simulink library "carnotUIBK"  (R2018b)
settings: Solver=VariableStepAuto  StartTime=0.0  StopTime=10.0  RelTol=1e-3  EnableMultiTasking=on
values from neighbouring files (symbols this model uses):
  A = 7*10*2    (= 140)    [theta_ground_v1.m]    (also in xlswrite1.m = num2cell(data))
  amb_factor = 1    [DOOR.m]    (also in WALL.m; WINDOW.m = 0)
  area = obj.width * obj.height    [DOOR.m]    (also in RES.m = []; ROOM.m = 0; THERMALZONE.m = area + room(kk).area; WALL.m = area - obj.doors(jj).calc_area())
  B = A/(0.5 * P)    (= 8.23529411765)    [theta_ground_v1.m]
  boundary = BOUNDARY()    [BUILDING.m]    (also in WALL.m = '')
  building = obj    [BUILDING.m]    (also in create_building_automatic.m = building.save(); ini_building_automatic.m = building.add_variant_hvac(building.variant_hvac, hvac); load_building_automatic.m = building.save())
  C = zeros(1,length(d)+1)    [CONSTRUCTION.m]    (also in DOOR.m = [0 0 0]; WALL.m = [0 0 0]; WINDOW.m = [0 0 0])
  control = 2    [GAIN.m]    (also in GAINS.m)
  cp = str2num(value)    [CONSTRUCTION.m]
  height = 0    [DOOR.m]    (also in ROOM.m; THERMALZONE.m; WALL.m; WINDOW.m)
  p = [timevec_weather weather(:,12)]    [BOUNDARY.m]    (also in WEATHER.m = 0; init_carnotUIBK.m = cell2mat(carnotUIBKpaths(i,2)))
  rho = str2num(value)    [CONSTRUCTION.m]    (also in theta_ground_v1.m = 2000)
  type = 1    [CONSTRUCTION.m]    (also in GAINS.m = raw_moisture{ii,3}; STRUCTURE.m = 0)
  view_factor = 1    [DOOR.m]    (also in WINDOW.m = 0)
  wall = []    [ROOM.m]
  z = obj.Z    [WALL.m]    (also in theta_ground_v1.m = 0)
  zone = obj.zone(ind)    [THERMALZONE.m]
undefined symbols (not defined in the file or in its folder): const, Dd, get_building, pos, Qdot_C, Qdot_H, Qdot_I_electricity, Qdot_I_light, Qdot_I_person, Qdot_S, Qdot_T_ground, Qdot_T_neighbour, Qdot_T_opaque, Qdot_T_window, Qdot_V_infiltration, Qdot_V_mech, Qdot_V_window, r_frame, solar_ratio, solar_ratio1, solar_ratio2, Tc, Tr, Ts, Uvalue, wallsurface, window, window_height, window_heigth, window_width, windowsurface, x_CO2, x_H2O, x_VOC
libraries: carnot x104, simulink x16, $bdroot x16, simulink_extras x14
(part 9 of 12)

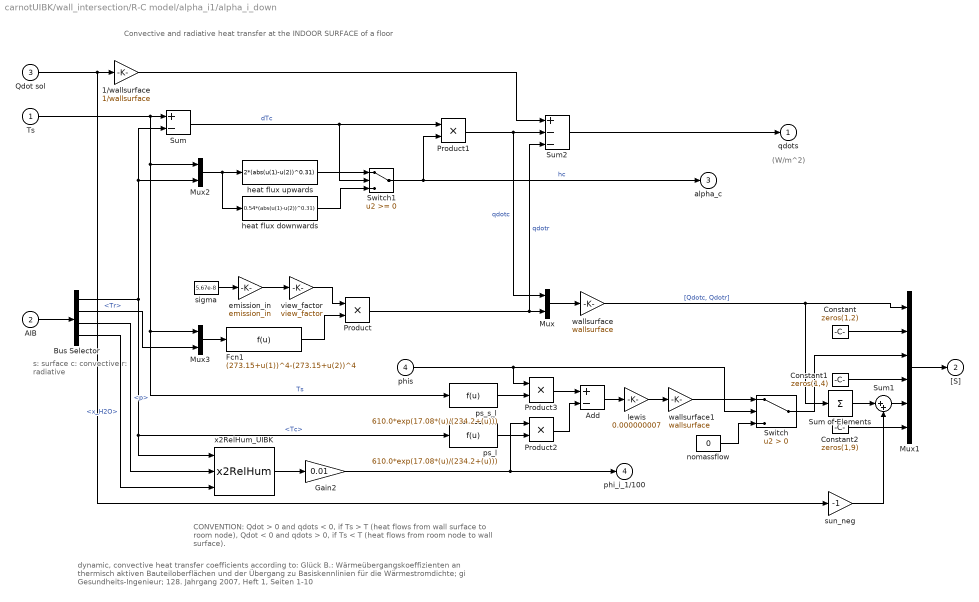
== system carnotUIBK/wall_intersection/R-C model/alpha_i1/alpha_i_down ==
  note: dynamic, convective heat transfer coefficients according to: Glück B.: Wärmeübergangskoeffizienten an thermisch aktiven Bauteiloberflächen
      | und der Übergang zu Basiskennlinien für die Wärmestromdichte; gi Gesundheits-Ingenieur; 128. Jahrgang 2007, Heft 1, Seiten 1-10
  note: s: surface
      | c: convective
      | r: radiative
  note: CONVENTION:
      | Qdot > 0 and qdots < 0, if Ts > T (heat flows from wall surface to room node),
      | Qdot < 0 and qdots > 0, if Ts < T (heat flows from room node to wall surface).
  note: Convective and radiative heat transfer at the INDOOR SURFACE of a floor
  note: (W/m^2)
  Ts : Inport
  AIB : Inport  Port=2
  Qdot sol : Inport  Port=3
  phis : Inport  Port=4
  1/wallsurface : Gain  Gain=1/wallsurface  SaturateOnIntegerOverflow=on  OutDataTypeStr=Inherit: Same as input  ParamDataTypeStr=Inherit: Same as input
  Add : Sum  Inputs=+-
  Bus Selector : BusSelector  OutputSignals=Tc,Tr,p,x_H2O
  Constant : Constant  Value=zeros(1,2)
  Constant1 : Constant  Value=zeros(1,4)
  Constant2 : Constant  Value=zeros(1,9)
  Fcn1 : Fcn  Expr=(273.15+u(1))^4-(273.15+u(2))^4
  Gain2 : Gain  Gain=0.01
  Mux : Mux  Inputs=2
  Mux1 : Mux  Inputs=[2 2 1 4 1 9]
  Mux2 : Mux  Inputs=2
  Mux3 : Mux  Inputs=2
  Product : Product  SaturateOnIntegerOverflow=on  RndMeth=Zero  InputSameDT=on  OutDataTypeStr=Inherit: Same as first input
  Product1 : Product  SaturateOnIntegerOverflow=on  RndMeth=Zero  InputSameDT=on  OutDataTypeStr=Inherit: Same as first input
  Product2 : Product  RndMeth=Zero
  Product3 : Product  RndMeth=Zero
  Sum : Sum  Inputs=+-  SaturateOnIntegerOverflow=on  InputSameDT=on  OutDataTypeStr=Inherit: Same as first input
  Sum of Elements : Sum  Inputs=+
  Sum1 : Sum  Inputs=|++
  Sum2 : Sum  Inputs=+--  SaturateOnIntegerOverflow=on  InputSameDT=on  OutDataTypeStr=Inherit: Same as first input
  Switch : Switch  Criteria=u2 > Threshold
  Switch1 : Switch
  emission_in : Gain  Gain=emission_in  SaturateOnIntegerOverflow=on  OutDataTypeStr=Inherit: Same as input  ParamDataTypeStr=Inherit: Same as input
  heat flux downwards : Fcn  Expr=0.54*(abs(u(1)-u(2))^0.31)
  heat flux upwards : Fcn  Expr=2*(abs(u(1)-u(2))^0.31)
  lewis : Gain  Gain=0.000000007  SaturateOnIntegerOverflow=on  OutDataTypeStr=Inherit: Same as input  ParamDataTypeStr=Inherit: Same as input
  nomassflow : Constant  Value=0
  ps_l : Fcn  Expr=610.0*exp(17.08*(u)/(234.2+(u)))
  ps_s_l : Fcn  Expr=610.0*exp(17.08*(u)/(234.2+(u)))
  sigma : Constant  Value=5.67e-8
  sun_neg : Gain  Gain=-1  SaturateOnIntegerOverflow=on  OutDataTypeStr=Inherit: Same as input  ParamDataTypeStr=Inherit: Same as input
  view_factor : Gain  Gain=view_factor  SaturateOnIntegerOverflow=on  OutDataTypeStr=Inherit: Same as input  ParamDataTypeStr=Inherit: Same as input
  wallsurface : Gain  Gain=wallsurface  SaturateOnIntegerOverflow=on  OutDataTypeStr=Inherit: Same as input  ParamDataTypeStr=Inherit: Same as input
  wallsurface1 : Gain  Gain=wallsurface  SaturateOnIntegerOverflow=on  OutDataTypeStr=Inherit: Same as input  ParamDataTypeStr=Inherit: Same as input
  x2RelHum_UIBK : carnot/Basic/Material_Properties/x2RelHum
  qdots : Outport  InitialOutput=0
  "[S]" : Outport  Port=2  InitialOutput=0
  alpha_c : Outport  Port=3  InitialOutput=0
  phi_i_1/100 : Outport  Port=4  InitialOutput=0
  wires:
  heat flux downwards/1 -> Switch1/3
  heat flux upwards/1 -> Switch1/1
  Sum/1 -> Product1/1, Switch1/2  "dTc"
  1/wallsurface/1 -> Sum2/1
  wallsurface/1 -> Sum of Elements/1, Mux1/1  "[Qdotc, Qdotr]"
  Switch1/1 -> alpha_c/1, Product1/2  "hc"
  Product1/1 -> Sum2/2, Mux/1  "qdotc"
  Mux2/1 -> heat flux upwards/1, heat flux downwards/1
  Bus Selector/2 -> Mux3/2  "<Tr>"
  Ts/1 -> Mux2/1, Mux3/1, ps_s_l/1, Sum/1  "Ts"
  Mux/1 -> wallsurface/1
  Product/1 -> Mux/2, Sum2/3  "qdotr"
  emission_in/1 -> view_factor/1
  Bus Selector/1 -> x2RelHum_UIBK/1, ps_l/1, Mux2/2, Sum/2  "<Tc>"
  AIB/1 -> Bus Selector/1
  Sum2/1 -> qdots/1
  Mux1/1 -> "[S]"/1
  sigma/1 -> emission_in/1
  Mux3/1 -> Fcn1/1
  Fcn1/1 -> Product/2
  x2RelHum_UIBK/1 -> Gain2/1
  Bus Selector/3 -> x2RelHum_UIBK/2  "<p>"
  Bus Selector/4 -> x2RelHum_UIBK/3  "<x_H2O>"
  Gain2/1 -> phi_i_1/100/1, Product2/1
  lewis/1 -> wallsurface1/1
  Constant2/1 -> Mux1/6
  Constant1/1 -> Mux1/4
  Constant/1 -> Mux1/2
  ps_l/1 -> Product2/2
  ps_s_l/1 -> Product3/2
  Product3/1 -> Add/1
  Product2/1 -> Add/2
  Add/1 -> lewis/1
  phis/1 -> Switch/2, Product3/1
  view_factor/1 -> Product/1
  wallsurface1/1 -> Switch/1
  Switch/1 -> Mux1/3
  nomassflow/1 -> Switch/3
  Sum1/1 -> Mux1/5
  Sum of Elements/1 -> Sum1/1
  Qdot sol/1 -> 1/wallsurface/1, sun_neg/1
  sun_neg/1 -> Sum1/2

== system carnotUIBK/wall_intersection/R-C model/alpha_i1/alpha_i_horizontal ==
  note: dynamic, convective heat transfer coefficients according to: Glück B.: Wärmeübergangskoeffizienten an thermisch aktiven Bauteiloberflächen
      | und der Übergang zu Basiskennlinien für die Wärmestromdichte; gi Gesundheits-Ingenieur; 128. Jahrgang 2007, Heft 1, Seiten 1-10
  note: s: surface
      | c: convective
      | r: radiative
  note: CONVENTION:
      | Qdot > 0 and qdots < 0, if Ts > T (heat flows from wall surface to room node),
      | Qdot < 0 and qdots > 0, if Ts < T (heat flows from room node to wall surface).
  note: Convective and radiative heat transfer at the INDOOR SURFACE of a VERTICAL OUTER WALL
  note: (W/m^2)
  Ts : Inport
  AIB : Inport  Port=2
  Qdot sol : Inport  Port=3
  phis : Inport  Port=4
  1/wallsurface : Gain  Gain=1/wallsurface  SaturateOnIntegerOverflow=on  OutDataTypeStr=Inherit: Same as input  ParamDataTypeStr=Inherit: Same as input
  Add : Sum  Inputs=+-
  Bus Selector : BusSelector  OutputSignals=Tc,Tr,p,x_H2O
  Constant : Constant  Value=zeros(1,2)
  Constant4 : Constant  Value=zeros(1,4)
  Constant5 : Constant  Value=zeros(1,9)
  Fcn : Fcn  Expr=1.6*(abs(u(1)-u(2)))^0.3
  Fcn1 : Fcn  Expr=(273.15+u(1))^4-(273.15+u(2))^4
  Gain2 : Gain  Gain=0.01
  Mux : Mux  Inputs=2
  Mux2 : Mux  Inputs=2
  Mux3 : Mux  Inputs=2
  Mux4 : Mux  Inputs=[2 2 1 4 1 9]
  Product : Product  SaturateOnIntegerOverflow=on  RndMeth=Zero  InputSameDT=on  OutDataTypeStr=Inherit: Same as first input
  Product1 : Product  SaturateOnIntegerOverflow=on  RndMeth=Zero  InputSameDT=on  OutDataTypeStr=Inherit: Same as first input
  Product2 : Product  RndMeth=Zero
  Product3 : Product  RndMeth=Zero
  Sum : Sum  Inputs=+-  SaturateOnIntegerOverflow=on  InputSameDT=on  OutDataTypeStr=Inherit: Same as first input
  Sum of Elements : Sum  Inputs=+
  Sum1 : Sum  Inputs=|++
  Sum2 : Sum  Inputs=+--  SaturateOnIntegerOverflow=on  InputSameDT=on  OutDataTypeStr=Inherit: Same as first input
  Switch : Switch  Criteria=u2 > Threshold
  emission_in : Gain  Gain=emission_in  SaturateOnIntegerOverflow=on  OutDataTypeStr=Inherit: Same as input  ParamDataTypeStr=Inherit: Same as input
  lewis : Gain  Gain=0.000000007  SaturateOnIntegerOverflow=on  OutDataTypeStr=Inherit: Same as input  ParamDataTypeStr=Inherit: Same as input
  nomassflow : Constant  Value=0
  ps_l : Fcn  Expr=610.0*exp(17.08*(u)/(234.2+(u)))
  ps_s_l : Fcn  Expr=610.0*exp(17.08*(u)/(234.2+(u)))
  sigma : Constant  Value=5.67e-8
  sun_neg : Gain  Gain=-1  SaturateOnIntegerOverflow=on  OutDataTypeStr=Inherit: Same as input  ParamDataTypeStr=Inherit: Same as input
  view_factor : Gain  Gain=view_factor  SaturateOnIntegerOverflow=on  OutDataTypeStr=Inherit: Same as input  ParamDataTypeStr=Inherit: Same as input
  wallsurface : Gain  Gain=wallsurface  SaturateOnIntegerOverflow=on  OutDataTypeStr=Inherit: Same as input  ParamDataTypeStr=Inherit: Same as input
  wallsurface1 : Gain  Gain=wallsurface  SaturateOnIntegerOverflow=on  OutDataTypeStr=Inherit: Same as input  ParamDataTypeStr=Inherit: Same as input
  x2RelHum_UIBK : carnot/Basic/Material_Properties/x2RelHum
  qdots : Outport  InitialOutput=0
  "[S]" : Outport  Port=2  InitialOutput=0
  alpha_c : Outport  Port=3  InitialOutput=0
  phi_i_1/100 : Outport  Port=4  InitialOutput=0
  wires:
  1/wallsurface/1 -> Sum2/1
  Qdot sol/1 -> sun_neg/1, 1/wallsurface/1
  wallsurface/1 -> Sum of Elements/1, Mux4/1  "[Qdotc, Qdotr]"
  Fcn/1 -> Product1/2, alpha_c/1  "hc"
  Product1/1 -> Sum2/2, Mux/1  "qdotc"
  Mux2/1 -> Fcn/1
  Bus Selector/2 -> Mux3/2  "<Tr>"
  Sum/1 -> Product1/1  "dTc"
  Ts/1 -> Mux2/1, Mux3/1, ps_s_l/1, Sum/1  "Ts"
  Mux/1 -> wallsurface/1
  Product/1 -> Mux/2, Sum2/3  "qdotr"
  emission_in/1 -> view_factor/1
  Bus Selector/1 -> x2RelHum_UIBK/1, ps_l/1, Mux2/2, Sum/2  "<Tc>"
  AIB/1 -> Bus Selector/1
  Sum2/1 -> qdots/1
  Mux4/1 -> "[S]"/1
  sigma/1 -> emission_in/1
  Mux3/1 -> Fcn1/1
  Fcn1/1 -> Product/2
  x2RelHum_UIBK/1 -> Gain2/1
  Bus Selector/3 -> x2RelHum_UIBK/2  "<p>"
  Bus Selector/4 -> x2RelHum_UIBK/3  "<x_H2O>"
  Gain2/1 -> phi_i_1/100/1, Product2/1
  lewis/1 -> wallsurface1/1
  ps_l/1 -> Product2/2
  ps_s_l/1 -> Product3/2
  Product3/1 -> Add/1
  Product2/1 -> Add/2
  Add/1 -> lewis/1
  phis/1 -> Switch/2, Product3/1
  view_factor/1 -> Product/1
  wallsurface1/1 -> Switch/1
  Switch/1 -> Mux4/3
  nomassflow/1 -> Switch/3
  Constant/1 -> Mux4/2
  Constant5/1 -> Mux4/6
  Constant4/1 -> Mux4/4
  Sum1/1 -> Mux4/5
  Sum of Elements/1 -> Sum1/1
  sun_neg/1 -> Sum1/2

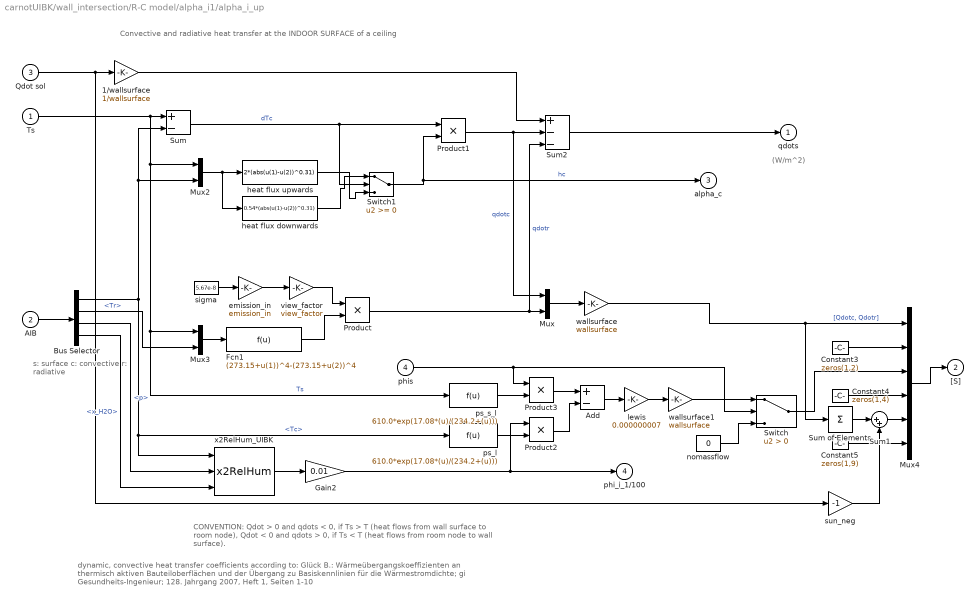
== system carnotUIBK/wall_intersection/R-C model/alpha_i1/alpha_i_up ==
  note: dynamic, convective heat transfer coefficients according to: Glück B.: Wärmeübergangskoeffizienten an thermisch aktiven Bauteiloberflächen
      | und der Übergang zu Basiskennlinien für die Wärmestromdichte; gi Gesundheits-Ingenieur; 128. Jahrgang 2007, Heft 1, Seiten 1-10
  note: s: surface
      | c: convective
      | r: radiative
  note: CONVENTION:
      | Qdot > 0 and qdots < 0, if Ts > T (heat flows from wall surface to room node),
      | Qdot < 0 and qdots > 0, if Ts < T (heat flows from room node to wall surface).
  note: Convective and radiative heat transfer at the INDOOR SURFACE of a ceiling
  note: (W/m^2)
  Ts : Inport
  AIB : Inport  Port=2
  Qdot sol : Inport  Port=3
  phis : Inport  Port=4
  1/wallsurface : Gain  Gain=1/wallsurface  SaturateOnIntegerOverflow=on  OutDataTypeStr=Inherit: Same as input  ParamDataTypeStr=Inherit: Same as input
  Add : Sum  Inputs=+-
  Bus Selector : BusSelector  OutputSignals=Tc,Tr,p,x_H2O
  Constant3 : Constant  Value=zeros(1,2)
  Constant4 : Constant  Value=zeros(1,4)
  Constant5 : Constant  Value=zeros(1,9)
  Fcn1 : Fcn  Expr=(273.15+u(1))^4-(273.15+u(2))^4
  Gain2 : Gain  Gain=0.01
  Mux : Mux  Inputs=2
  Mux2 : Mux  Inputs=2
  Mux3 : Mux  Inputs=2
  Mux4 : Mux  Inputs=[2 2 1 4 1 9]
  Product : Product  SaturateOnIntegerOverflow=on  RndMeth=Zero  InputSameDT=on  OutDataTypeStr=Inherit: Same as first input
  Product1 : Product  SaturateOnIntegerOverflow=on  RndMeth=Zero  InputSameDT=on  OutDataTypeStr=Inherit: Same as first input
  Product2 : Product  RndMeth=Zero
  Product3 : Product  RndMeth=Zero
  Sum : Sum  Inputs=+-  SaturateOnIntegerOverflow=on  InputSameDT=on  OutDataTypeStr=Inherit: Same as first input
  Sum of Elements : Sum  Inputs=+
  Sum1 : Sum  Inputs=|++
  Sum2 : Sum  Inputs=+--  SaturateOnIntegerOverflow=on  InputSameDT=on  OutDataTypeStr=Inherit: Same as first input
  Switch : Switch  Criteria=u2 > Threshold
  Switch1 : Switch
  emission_in : Gain  Gain=emission_in  SaturateOnIntegerOverflow=on  OutDataTypeStr=Inherit: Same as input  ParamDataTypeStr=Inherit: Same as input
  heat flux downwards : Fcn  Expr=0.54*(abs(u(1)-u(2))^0.31)
  heat flux upwards : Fcn  Expr=2*(abs(u(1)-u(2))^0.31)
  lewis : Gain  Gain=0.000000007  SaturateOnIntegerOverflow=on  OutDataTypeStr=Inherit: Same as input  ParamDataTypeStr=Inherit: Same as input
  nomassflow : Constant  Value=0
  ps_l : Fcn  Expr=610.0*exp(17.08*(u)/(234.2+(u)))
  ps_s_l : Fcn  Expr=610.0*exp(17.08*(u)/(234.2+(u)))
  sigma : Constant  Value=5.67e-8
  sun_neg : Gain  Gain=-1  SaturateOnIntegerOverflow=on  OutDataTypeStr=Inherit: Same as input  ParamDataTypeStr=Inherit: Same as input
  view_factor : Gain  Gain=view_factor  SaturateOnIntegerOverflow=on  OutDataTypeStr=Inherit: Same as input  ParamDataTypeStr=Inherit: Same as input
  wallsurface : Gain  Gain=wallsurface  SaturateOnIntegerOverflow=on  OutDataTypeStr=Inherit: Same as input  ParamDataTypeStr=Inherit: Same as input
  wallsurface1 : Gain  Gain=wallsurface  SaturateOnIntegerOverflow=on  OutDataTypeStr=Inherit: Same as input  ParamDataTypeStr=Inherit: Same as input
  x2RelHum_UIBK : carnot/Basic/Material_Properties/x2RelHum
  qdots : Outport  InitialOutput=0
  "[S]" : Outport  Port=2  InitialOutput=0
  alpha_c : Outport  Port=3  InitialOutput=0
  phi_i_1/100 : Outport  Port=4  InitialOutput=0
  wires:
  heat flux downwards/1 -> Switch1/1
  heat flux upwards/1 -> Switch1/3
  Sum/1 -> Product1/1, Switch1/2  "dTc"
  1/wallsurface/1 -> Sum2/1
  Qdot sol/1 -> sun_neg/1, 1/wallsurface/1
  Switch1/1 -> alpha_c/1, Product1/2  "hc"
  Product1/1 -> Sum2/2, Mux/1  "qdotc"
  Mux2/1 -> heat flux upwards/1, heat flux downwards/1
  Bus Selector/2 -> Mux3/2  "<Tr>"
  Ts/1 -> Mux2/1, Mux3/1, ps_s_l/1, Sum/1  "Ts"
  Mux/1 -> wallsurface/1
  Product/1 -> Mux/2, Sum2/3  "qdotr"
  emission_in/1 -> view_factor/1
  Bus Selector/1 -> x2RelHum_UIBK/1, ps_l/1, Mux2/2, Sum/2  "<Tc>"
  AIB/1 -> Bus Selector/1
  Sum2/1 -> qdots/1
  sigma/1 -> emission_in/1
  Mux3/1 -> Fcn1/1
  Fcn1/1 -> Product/2
  x2RelHum_UIBK/1 -> Gain2/1
  Bus Selector/3 -> x2RelHum_UIBK/2  "<p>"
  Bus Selector/4 -> x2RelHum_UIBK/3  "<x_H2O>"
  Gain2/1 -> phi_i_1/100/1, Product2/1
  lewis/1 -> wallsurface1/1
  ps_l/1 -> Product2/2
  ps_s_l/1 -> Product3/2
  Product3/1 -> Add/1
  Product2/1 -> Add/2
  Add/1 -> lewis/1
  phis/1 -> Switch/2, Product3/1
  view_factor/1 -> Product/1
  wallsurface1/1 -> Switch/1
  Switch/1 -> Mux4/3
  nomassflow/1 -> Switch/3
  wallsurface/1 -> Sum of Elements/1, Mux4/1  "[Qdotc, Qdotr]"
  Mux4/1 -> "[S]"/1
  Constant5/1 -> Mux4/6
  Constant4/1 -> Mux4/4
  Constant3/1 -> Mux4/2
  Sum of Elements/1 -> Sum1/1
  Sum1/1 -> Mux4/5
  sun_neg/1 -> Sum1/2

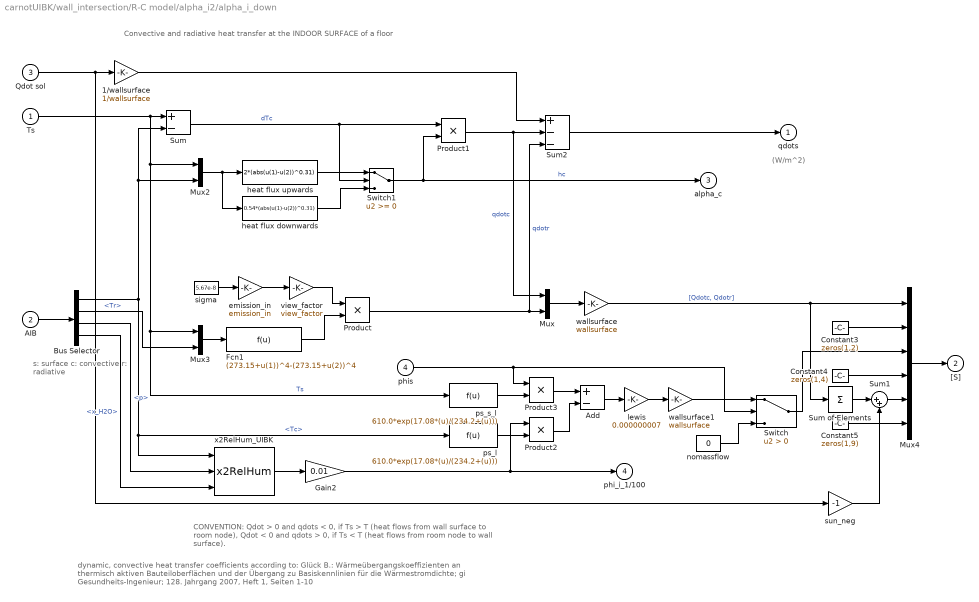
== system carnotUIBK/wall_intersection/R-C model/alpha_i2/alpha_i_down ==
  note: (W/m^2)
  note: Convective and radiative heat transfer at the INDOOR SURFACE of a floor
  note: CONVENTION:
      | Qdot > 0 and qdots < 0, if Ts > T (heat flows from wall surface to room node),
      | Qdot < 0 and qdots > 0, if Ts < T (heat flows from room node to wall surface).
  note: s: surface
      | c: convective
      | r: radiative
  note: dynamic, convective heat transfer coefficients according to: Glück B.: Wärmeübergangskoeffizienten an thermisch aktiven Bauteiloberflächen
      | und der Übergang zu Basiskennlinien für die Wärmestromdichte; gi Gesundheits-Ingenieur; 128. Jahrgang 2007, Heft 1, Seiten 1-10
  Ts : Inport
  AIB : Inport  Port=2
  Qdot sol : Inport  Port=3
  phis : Inport  Port=4
  1/wallsurface : Gain  Gain=1/wallsurface  SaturateOnIntegerOverflow=on  OutDataTypeStr=Inherit: Same as input  ParamDataTypeStr=Inherit: Same as input
  Add : Sum  Inputs=+-
  Bus Selector : BusSelector  OutputSignals=Tc,Tr,p,x_H2O
  Constant3 : Constant  Value=zeros(1,2)
  Constant4 : Constant  Value=zeros(1,4)
  Constant5 : Constant  Value=zeros(1,9)
  Fcn1 : Fcn  Expr=(273.15+u(1))^4-(273.15+u(2))^4
  Gain2 : Gain  Gain=0.01
  Mux : Mux  Inputs=2
  Mux2 : Mux  Inputs=2
  Mux3 : Mux  Inputs=2
  Mux4 : Mux  Inputs=[2 2 1 4 1 9]
  Product : Product  SaturateOnIntegerOverflow=on  RndMeth=Zero  InputSameDT=on  OutDataTypeStr=Inherit: Same as first input
  Product1 : Product  SaturateOnIntegerOverflow=on  RndMeth=Zero  InputSameDT=on  OutDataTypeStr=Inherit: Same as first input
  Product2 : Product  RndMeth=Zero
  Product3 : Product  RndMeth=Zero
  Sum : Sum  Inputs=+-  SaturateOnIntegerOverflow=on  InputSameDT=on  OutDataTypeStr=Inherit: Same as first input
  Sum of Elements : Sum  Inputs=+
  Sum1 : Sum  Inputs=|++
  Sum2 : Sum  Inputs=+--  SaturateOnIntegerOverflow=on  InputSameDT=on  OutDataTypeStr=Inherit: Same as first input
  Switch : Switch  Criteria=u2 > Threshold
  Switch1 : Switch
  emission_in : Gain  Gain=emission_in  SaturateOnIntegerOverflow=on  OutDataTypeStr=Inherit: Same as input  ParamDataTypeStr=Inherit: Same as input
  heat flux downwards : Fcn  Expr=0.54*(abs(u(1)-u(2))^0.31)
  heat flux upwards : Fcn  Expr=2*(abs(u(1)-u(2))^0.31)
  lewis : Gain  Gain=0.000000007  SaturateOnIntegerOverflow=on  OutDataTypeStr=Inherit: Same as input  ParamDataTypeStr=Inherit: Same as input
  nomassflow : Constant  Value=0
  ps_l : Fcn  Expr=610.0*exp(17.08*(u)/(234.2+(u)))
  ps_s_l : Fcn  Expr=610.0*exp(17.08*(u)/(234.2+(u)))
  sigma : Constant  Value=5.67e-8
  sun_neg : Gain  Gain=-1  SaturateOnIntegerOverflow=on  OutDataTypeStr=Inherit: Same as input  ParamDataTypeStr=Inherit: Same as input
  view_factor : Gain  Gain=view_factor  SaturateOnIntegerOverflow=on  OutDataTypeStr=Inherit: Same as input  ParamDataTypeStr=Inherit: Same as input
  wallsurface : Gain  Gain=wallsurface  SaturateOnIntegerOverflow=on  OutDataTypeStr=Inherit: Same as input  ParamDataTypeStr=Inherit: Same as input
  wallsurface1 : Gain  Gain=wallsurface  SaturateOnIntegerOverflow=on  OutDataTypeStr=Inherit: Same as input  ParamDataTypeStr=Inherit: Same as input
  x2RelHum_UIBK : carnot/Basic/Material_Properties/x2RelHum
  qdots : Outport  InitialOutput=0
  "[S]" : Outport  Port=2  InitialOutput=0
  alpha_c : Outport  Port=3  InitialOutput=0
  phi_i_1/100 : Outport  Port=4  InitialOutput=0
  wires:
  nomassflow/1 -> Switch/3
  Switch/1 -> Mux4/3
  wallsurface1/1 -> Switch/1
  view_factor/1 -> Product/1
  phis/1 -> Product3/1, Switch/2
  Add/1 -> lewis/1
  Product2/1 -> Add/2
  Product3/1 -> Add/1
  ps_s_l/1 -> Product3/2
  ps_l/1 -> Product2/2
  lewis/1 -> wallsurface1/1
  Gain2/1 -> Product2/1, phi_i_1/100/1
  Bus Selector/4 -> x2RelHum_UIBK/3  "<x_H2O>"
  Bus Selector/3 -> x2RelHum_UIBK/2  "<p>"
  x2RelHum_UIBK/1 -> Gain2/1
  Fcn1/1 -> Product/2
  Mux3/1 -> Fcn1/1
  sigma/1 -> emission_in/1
  Mux4/1 -> "[S]"/1
  Sum2/1 -> qdots/1
  AIB/1 -> Bus Selector/1
  Bus Selector/1 -> Sum/2, Mux2/2, x2RelHum_UIBK/1, ps_l/1  "<Tc>"
  emission_in/1 -> view_factor/1
  Product/1 -> Sum2/3, Mux/2  "qdotr"
  Mux/1 -> wallsurface/1
  Ts/1 -> Sum/1, ps_s_l/1, Mux3/1, Mux2/1  "Ts"
  Bus Selector/2 -> Mux3/2  "<Tr>"
  Mux2/1 -> heat flux downwards/1, heat flux upwards/1
  Product1/1 -> Mux/1, Sum2/2  "qdotc"
  Switch1/1 -> Product1/2, alpha_c/1  "hc"
  wallsurface/1 -> Sum of Elements/1, Mux4/1  "[Qdotc, Qdotr]"
  Qdot sol/1 -> sun_neg/1, 1/wallsurface/1
  1/wallsurface/1 -> Sum2/1
  Sum/1 -> Switch1/2, Product1/1  "dTc"
  heat flux upwards/1 -> Switch1/1
  heat flux downwards/1 -> Switch1/3
  Constant5/1 -> Mux4/6
  Constant4/1 -> Mux4/4
  Constant3/1 -> Mux4/2
  Sum of Elements/1 -> Sum1/1
  Sum1/1 -> Mux4/5
  sun_neg/1 -> Sum1/2

== system carnotUIBK/wall_intersection/R-C model/alpha_i2/alpha_i_horizontal ==
  note: (W/m^2)
  note: Convective and radiative heat transfer at the INDOOR SURFACE of a VERTICAL OUTER WALL
  note: CONVENTION:
      | Qdot > 0 and qdots < 0, if Ts > T (heat flows from wall surface to room node),
      | Qdot < 0 and qdots > 0, if Ts < T (heat flows from room node to wall surface).
  note: s: surface
      | c: convective
      | r: radiative
  note: dynamic, convective heat transfer coefficients according to: Glück B.: Wärmeübergangskoeffizienten an thermisch aktiven Bauteiloberflächen
      | und der Übergang zu Basiskennlinien für die Wärmestromdichte; gi Gesundheits-Ingenieur; 128. Jahrgang 2007, Heft 1, Seiten 1-10
  Ts : Inport
  AIB : Inport  Port=2
  Qdot sol : Inport  Port=3
  phis : Inport  Port=4
  1/wallsurface : Gain  Gain=1/wallsurface  SaturateOnIntegerOverflow=on  OutDataTypeStr=Inherit: Same as input  ParamDataTypeStr=Inherit: Same as input
  Add : Sum  Inputs=+-
  Bus Selector : BusSelector  OutputSignals=Tc,Tr,p,x_H2O
  Constant3 : Constant  Value=zeros(1,2)
  Constant4 : Constant  Value=zeros(1,4)
  Constant5 : Constant  Value=zeros(1,9)
  Fcn : Fcn  Expr=1.6*(abs(u(1)-u(2)))^0.3
  Fcn1 : Fcn  Expr=(273.15+u(1))^4-(273.15+u(2))^4
  Gain2 : Gain  Gain=0.01
  Mux : Mux  Inputs=2
  Mux2 : Mux  Inputs=2
  Mux3 : Mux  Inputs=2
  Mux4 : Mux  Inputs=[2 2 1 4 1 9]
  Product : Product  SaturateOnIntegerOverflow=on  RndMeth=Zero  InputSameDT=on  OutDataTypeStr=Inherit: Same as first input
  Product1 : Product  SaturateOnIntegerOverflow=on  RndMeth=Zero  InputSameDT=on  OutDataTypeStr=Inherit: Same as first input
  Product2 : Product  RndMeth=Zero
  Product3 : Product  RndMeth=Zero
  Sum : Sum  Inputs=+-  SaturateOnIntegerOverflow=on  InputSameDT=on  OutDataTypeStr=Inherit: Same as first input
  Sum of Elements : Sum  Inputs=+
  Sum1 : Sum  Inputs=|++
  Sum2 : Sum  Inputs=+--  SaturateOnIntegerOverflow=on  InputSameDT=on  OutDataTypeStr=Inherit: Same as first input
  Switch : Switch  Criteria=u2 > Threshold
  emission_in : Gain  Gain=emission_in  SaturateOnIntegerOverflow=on  OutDataTypeStr=Inherit: Same as input  ParamDataTypeStr=Inherit: Same as input
  lewis : Gain  Gain=0.000000007  SaturateOnIntegerOverflow=on  OutDataTypeStr=Inherit: Same as input  ParamDataTypeStr=Inherit: Same as input
  nomassflow : Constant  Value=0
  ps_l : Fcn  Expr=610.0*exp(17.08*(u)/(234.2+(u)))
  ps_s_l : Fcn  Expr=610.0*exp(17.08*(u)/(234.2+(u)))
  sigma : Constant  Value=5.67e-8
  sun_neg : Gain  Gain=-1  SaturateOnIntegerOverflow=on  OutDataTypeStr=Inherit: Same as input  ParamDataTypeStr=Inherit: Same as input
  view_factor : Gain  Gain=view_factor  SaturateOnIntegerOverflow=on  OutDataTypeStr=Inherit: Same as input  ParamDataTypeStr=Inherit: Same as input
  wallsurface : Gain  Gain=wallsurface  SaturateOnIntegerOverflow=on  OutDataTypeStr=Inherit: Same as input  ParamDataTypeStr=Inherit: Same as input
  wallsurface1 : Gain  Gain=wallsurface  SaturateOnIntegerOverflow=on  OutDataTypeStr=Inherit: Same as input  ParamDataTypeStr=Inherit: Same as input
  x2RelHum_UIBK : carnot/Basic/Material_Properties/x2RelHum
  qdots : Outport  InitialOutput=0
  "[S]" : Outport  Port=2  InitialOutput=0
  alpha_c : Outport  Port=3  InitialOutput=0
  phi_i_1/100 : Outport  Port=4  InitialOutput=0
  wires:
  nomassflow/1 -> Switch/3
  Switch/1 -> Mux4/3
  wallsurface1/1 -> Switch/1
  view_factor/1 -> Product/1
  phis/1 -> Product3/1, Switch/2
  Add/1 -> lewis/1
  Product2/1 -> Add/2
  Product3/1 -> Add/1
  ps_s_l/1 -> Product3/2
  ps_l/1 -> Product2/2
  lewis/1 -> wallsurface1/1
  Gain2/1 -> Product2/1, phi_i_1/100/1
  Bus Selector/4 -> x2RelHum_UIBK/3  "<x_H2O>"
  Bus Selector/3 -> x2RelHum_UIBK/2  "<p>"
  x2RelHum_UIBK/1 -> Gain2/1
  Fcn1/1 -> Product/2
  Mux3/1 -> Fcn1/1
  sigma/1 -> emission_in/1
  Mux4/1 -> "[S]"/1
  Sum2/1 -> qdots/1
  AIB/1 -> Bus Selector/1
  Bus Selector/1 -> Sum/2, Mux2/2, x2RelHum_UIBK/1, ps_l/1  "<Tc>"
  emission_in/1 -> view_factor/1
  Product/1 -> Sum2/3, Mux/2  "qdotr"
  Mux/1 -> wallsurface/1
  Ts/1 -> Sum/1, ps_s_l/1, Mux3/1, Mux2/1  "Ts"
  Sum/1 -> Product1/1  "dTc"
  Bus Selector/2 -> Mux3/2  "<Tr>"
  Mux2/1 -> Fcn/1
  Product1/1 -> Mux/1, Sum2/2  "qdotc"
  Fcn/1 -> alpha_c/1, Product1/2  "hc"
  wallsurface/1 -> Sum of Elements/1, Mux4/1  "[Qdotc, Qdotr]"
  Qdot sol/1 -> sun_neg/1, 1/wallsurface/1
  1/wallsurface/1 -> Sum2/1
  Constant5/1 -> Mux4/6
  Constant4/1 -> Mux4/4
  Constant3/1 -> Mux4/2
  Sum of Elements/1 -> Sum1/1
  Sum1/1 -> Mux4/5
  sun_neg/1 -> Sum1/2

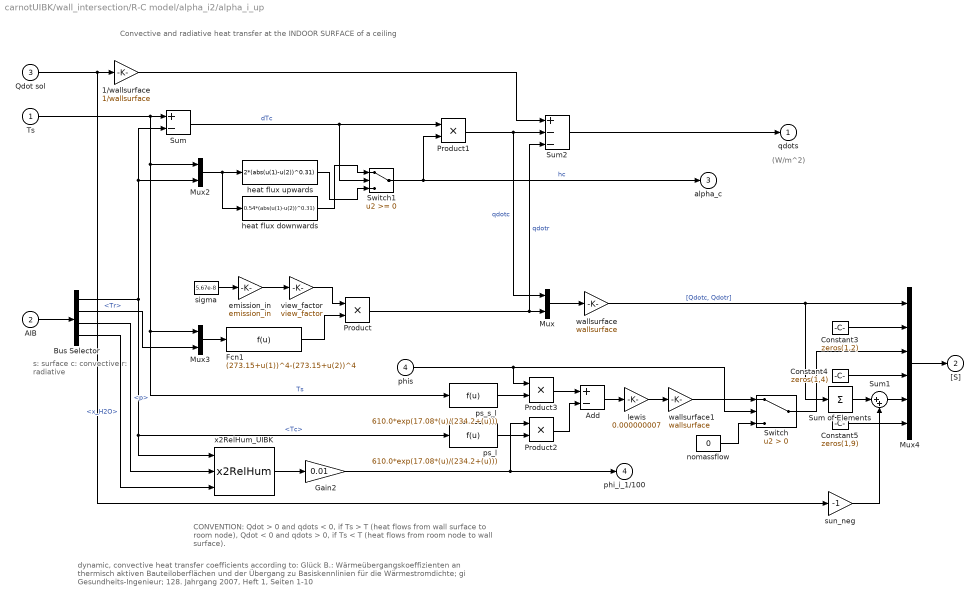
== system carnotUIBK/wall_intersection/R-C model/alpha_i2/alpha_i_up ==
  note: (W/m^2)
  note: Convective and radiative heat transfer at the INDOOR SURFACE of a ceiling
  note: CONVENTION:
      | Qdot > 0 and qdots < 0, if Ts > T (heat flows from wall surface to room node),
      | Qdot < 0 and qdots > 0, if Ts < T (heat flows from room node to wall surface).
  note: s: surface
      | c: convective
      | r: radiative
  note: dynamic, convective heat transfer coefficients according to: Glück B.: Wärmeübergangskoeffizienten an thermisch aktiven Bauteiloberflächen
      | und der Übergang zu Basiskennlinien für die Wärmestromdichte; gi Gesundheits-Ingenieur; 128. Jahrgang 2007, Heft 1, Seiten 1-10
  Ts : Inport
  AIB : Inport  Port=2
  Qdot sol : Inport  Port=3
  phis : Inport  Port=4
  1/wallsurface : Gain  Gain=1/wallsurface  SaturateOnIntegerOverflow=on  OutDataTypeStr=Inherit: Same as input  ParamDataTypeStr=Inherit: Same as input
  Add : Sum  Inputs=+-
  Bus Selector : BusSelector  OutputSignals=Tc,Tr,p,x_H2O
  Constant3 : Constant  Value=zeros(1,2)
  Constant4 : Constant  Value=zeros(1,4)
  Constant5 : Constant  Value=zeros(1,9)
  Fcn1 : Fcn  Expr=(273.15+u(1))^4-(273.15+u(2))^4
  Gain2 : Gain  Gain=0.01
  Mux : Mux  Inputs=2
  Mux2 : Mux  Inputs=2
  Mux3 : Mux  Inputs=2
  Mux4 : Mux  Inputs=[2 2 1 4 1 9]
  Product : Product  SaturateOnIntegerOverflow=on  RndMeth=Zero  InputSameDT=on  OutDataTypeStr=Inherit: Same as first input
  Product1 : Product  SaturateOnIntegerOverflow=on  RndMeth=Zero  InputSameDT=on  OutDataTypeStr=Inherit: Same as first input
  Product2 : Product  RndMeth=Zero
  Product3 : Product  RndMeth=Zero
  Sum : Sum  Inputs=+-  SaturateOnIntegerOverflow=on  InputSameDT=on  OutDataTypeStr=Inherit: Same as first input
  Sum of Elements : Sum  Inputs=+
  Sum1 : Sum  Inputs=|++
  Sum2 : Sum  Inputs=+--  SaturateOnIntegerOverflow=on  InputSameDT=on  OutDataTypeStr=Inherit: Same as first input
  Switch : Switch  Criteria=u2 > Threshold
  Switch1 : Switch
  emission_in : Gain  Gain=emission_in  SaturateOnIntegerOverflow=on  OutDataTypeStr=Inherit: Same as input  ParamDataTypeStr=Inherit: Same as input
  heat flux downwards : Fcn  Expr=0.54*(abs(u(1)-u(2))^0.31)
  heat flux upwards : Fcn  Expr=2*(abs(u(1)-u(2))^0.31)
  lewis : Gain  Gain=0.000000007  SaturateOnIntegerOverflow=on  OutDataTypeStr=Inherit: Same as input  ParamDataTypeStr=Inherit: Same as input
  nomassflow : Constant  Value=0
  ps_l : Fcn  Expr=610.0*exp(17.08*(u)/(234.2+(u)))
  ps_s_l : Fcn  Expr=610.0*exp(17.08*(u)/(234.2+(u)))
  sigma : Constant  Value=5.67e-8
  sun_neg : Gain  Gain=-1  SaturateOnIntegerOverflow=on  OutDataTypeStr=Inherit: Same as input  ParamDataTypeStr=Inherit: Same as input
  view_factor : Gain  Gain=view_factor  SaturateOnIntegerOverflow=on  OutDataTypeStr=Inherit: Same as input  ParamDataTypeStr=Inherit: Same as input
  wallsurface : Gain  Gain=wallsurface  SaturateOnIntegerOverflow=on  OutDataTypeStr=Inherit: Same as input  ParamDataTypeStr=Inherit: Same as input
  wallsurface1 : Gain  Gain=wallsurface  SaturateOnIntegerOverflow=on  OutDataTypeStr=Inherit: Same as input  ParamDataTypeStr=Inherit: Same as input
  x2RelHum_UIBK : carnot/Basic/Material_Properties/x2RelHum
  qdots : Outport  InitialOutput=0
  "[S]" : Outport  Port=2  InitialOutput=0
  alpha_c : Outport  Port=3  InitialOutput=0
  phi_i_1/100 : Outport  Port=4  InitialOutput=0
  wires:
  nomassflow/1 -> Switch/3
  Switch/1 -> Mux4/3
  wallsurface1/1 -> Switch/1
  view_factor/1 -> Product/1
  phis/1 -> Product3/1, Switch/2
  Add/1 -> lewis/1
  Product2/1 -> Add/2
  Product3/1 -> Add/1
  ps_s_l/1 -> Product3/2
  ps_l/1 -> Product2/2
  lewis/1 -> wallsurface1/1
  Gain2/1 -> Product2/1, phi_i_1/100/1
  Bus Selector/4 -> x2RelHum_UIBK/3  "<x_H2O>"
  Bus Selector/3 -> x2RelHum_UIBK/2  "<p>"
  x2RelHum_UIBK/1 -> Gain2/1
  Fcn1/1 -> Product/2
  Mux3/1 -> Fcn1/1
  sigma/1 -> emission_in/1
  Mux4/1 -> "[S]"/1
  Sum2/1 -> qdots/1
  AIB/1 -> Bus Selector/1
  Bus Selector/1 -> Sum/2, Mux2/2, x2RelHum_UIBK/1, ps_l/1  "<Tc>"
  emission_in/1 -> view_factor/1
  Product/1 -> Sum2/3, Mux/2  "qdotr"
  Mux/1 -> wallsurface/1
  Ts/1 -> Sum/1, ps_s_l/1, Mux3/1, Mux2/1  "Ts"
  Bus Selector/2 -> Mux3/2  "<Tr>"
  Mux2/1 -> heat flux downwards/1, heat flux upwards/1
  Product1/1 -> Mux/1, Sum2/2  "qdotc"
  Switch1/1 -> Product1/2, alpha_c/1  "hc"
  wallsurface/1 -> Sum of Elements/1, Mux4/1  "[Qdotc, Qdotr]"
  Qdot sol/1 -> sun_neg/1, 1/wallsurface/1
  1/wallsurface/1 -> Sum2/1
  Sum/1 -> Switch1/2, Product1/1  "dTc"
  heat flux upwards/1 -> Switch1/3
  heat flux downwards/1 -> Switch1/1
  Constant5/1 -> Mux4/6
  Constant4/1 -> Mux4/4
  Constant3/1 -> Mux4/2
  Sum of Elements/1 -> Sum1/1
  Sum1/1 -> Mux4/5
  sun_neg/1 -> Sum1/2

== system carnotUIBK/wall_intersection/UA/Rsi/down ==
  0.17+0.10 : Constant  Value=0.27
  Rsi : Outport
  wires:
  0.17+0.10/1 -> Rsi/1

== system carnotUIBK/wall_intersection/UA/Rsi/horizontal ==
  2x0.13 : Constant  Value=0.26
  Rsi : Outport
  wires:
  2x0.13/1 -> Rsi/1

== system carnotUIBK/wall_intersection/UA/Rsi/up ==
  0.10+0.17 : Constant  Value=0.27
  Rsi : Outport
  wires:
  0.10+0.17/1 -> Rsi/1

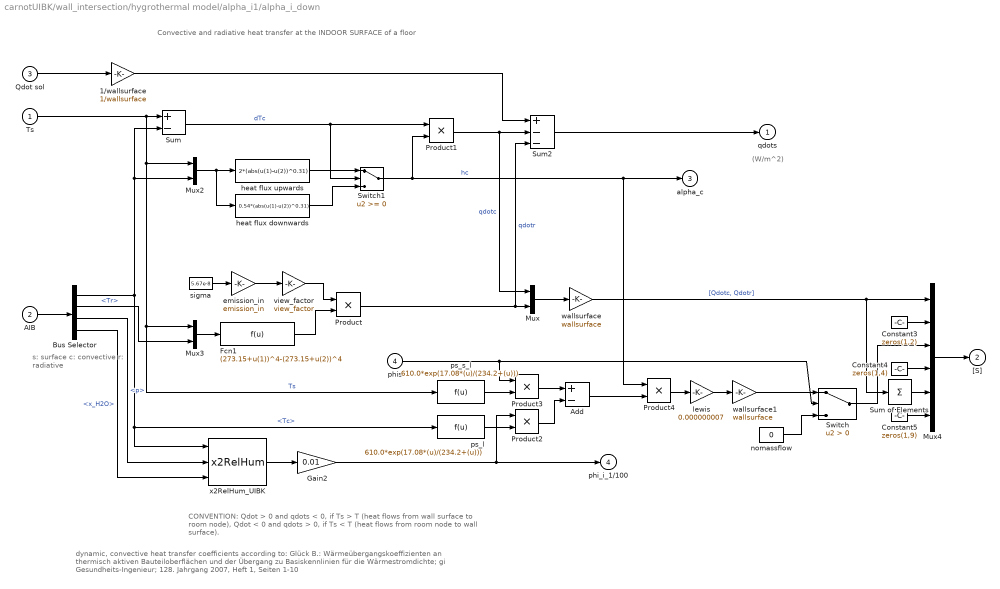
== system carnotUIBK/wall_intersection/hygrothermal model/alpha_i1/alpha_i_down ==
  note: dynamic, convective heat transfer coefficients according to: Glück B.: Wärmeübergangskoeffizienten an thermisch aktiven Bauteiloberflächen
      | und der Übergang zu Basiskennlinien für die Wärmestromdichte; gi Gesundheits-Ingenieur; 128. Jahrgang 2007, Heft 1, Seiten 1-10
  note: s: surface
      | c: convective
      | r: radiative
  note: CONVENTION:
      | Qdot > 0 and qdots < 0, if Ts > T (heat flows from wall surface to room node),
      | Qdot < 0 and qdots > 0, if Ts < T (heat flows from room node to wall surface).
  note: Convective and radiative heat transfer at the INDOOR SURFACE of a floor
  note: (W/m^2)
  Ts : Inport
  AIB : Inport  Port=2
  Qdot sol : Inport  Port=3
  phis : Inport  Port=4
  1/wallsurface : Gain  Gain=1/wallsurface  SaturateOnIntegerOverflow=on  OutDataTypeStr=Inherit: Same as input  ParamDataTypeStr=Inherit: Same as input
  Add : Sum  Inputs=+-
  Bus Selector : BusSelector  OutputSignals=Tc,Tr,p,x_H2O
  Constant3 : Constant  Value=zeros(1,2)
  Constant4 : Constant  Value=zeros(1,4)
  Constant5 : Constant  Value=zeros(1,9)
  Fcn1 : Fcn  Expr=(273.15+u(1))^4-(273.15+u(2))^4
  Gain2 : Gain  Gain=0.01
  Mux : Mux  Inputs=2
  Mux2 : Mux  Inputs=2
  Mux3 : Mux  Inputs=2
  Mux4 : Mux  Inputs=[2 2 1 4 1 9]
  Product : Product  SaturateOnIntegerOverflow=on  RndMeth=Zero  InputSameDT=on  OutDataTypeStr=Inherit: Same as first input
  Product1 : Product  SaturateOnIntegerOverflow=on  RndMeth=Zero  InputSameDT=on  OutDataTypeStr=Inherit: Same as first input
  Product2 : Product  RndMeth=Zero
  Product3 : Product  RndMeth=Zero
  Product4 : Product  SaturateOnIntegerOverflow=on  RndMeth=Zero  InputSameDT=on  OutDataTypeStr=Inherit: Same as first input
  Sum : Sum  Inputs=+-  SaturateOnIntegerOverflow=on  InputSameDT=on  OutDataTypeStr=Inherit: Same as first input
  Sum of Elements : Sum  Inputs=+
  Sum2 : Sum  Inputs=+--  SaturateOnIntegerOverflow=on  InputSameDT=on  OutDataTypeStr=Inherit: Same as first input
  Switch : Switch  Criteria=u2 > Threshold
  Switch1 : Switch
  emission_in : Gain  Gain=emission_in  SaturateOnIntegerOverflow=on  OutDataTypeStr=Inherit: Same as input  ParamDataTypeStr=Inherit: Same as input
  heat flux downwards : Fcn  Expr=0.54*(abs(u(1)-u(2))^0.31)
  heat flux upwards : Fcn  Expr=2*(abs(u(1)-u(2))^0.31)
  lewis : Gain  Gain=0.000000007  SaturateOnIntegerOverflow=on  OutDataTypeStr=Inherit: Same as input  ParamDataTypeStr=Inherit: Same as input
  nomassflow : Constant  Value=0
  ps_l : Fcn  Expr=610.0*exp(17.08*(u)/(234.2+(u)))
  ps_s_l : Fcn  Expr=610.0*exp(17.08*(u)/(234.2+(u)))
  sigma : Constant  Value=5.67e-8
  view_factor : Gain  Gain=view_factor  SaturateOnIntegerOverflow=on  OutDataTypeStr=Inherit: Same as input  ParamDataTypeStr=Inherit: Same as input
  wallsurface : Gain  Gain=wallsurface  SaturateOnIntegerOverflow=on  OutDataTypeStr=Inherit: Same as input  ParamDataTypeStr=Inherit: Same as input
  wallsurface1 : Gain  Gain=wallsurface  SaturateOnIntegerOverflow=on  OutDataTypeStr=Inherit: Same as input  ParamDataTypeStr=Inherit: Same as input
  x2RelHum_UIBK : carnot/Basic/Material_Properties/x2RelHum
  qdots : Outport  InitialOutput=0
  "[S]" : Outport  Port=2  InitialOutput=0
  alpha_c : Outport  Port=3  InitialOutput=0
  phi_i_1/100 : Outport  Port=4  InitialOutput=0
  wires:
  heat flux downwards/1 -> Switch1/3
  heat flux upwards/1 -> Switch1/1
  Sum/1 -> Product1/1, Switch1/2  "dTc"
  1/wallsurface/1 -> Sum2/1
  Qdot sol/1 -> 1/wallsurface/1
  wallsurface/1 -> Sum of Elements/1, Mux4/1  "[Qdotc, Qdotr]"
  Switch1/1 -> Product4/1, alpha_c/1, Product1/2  "hc"
  Product1/1 -> Sum2/2, Mux/1  "qdotc"
  Mux2/1 -> heat flux upwards/1, heat flux downwards/1
  Bus Selector/2 -> Mux3/2  "<Tr>"
  Ts/1 -> Mux2/1, Mux3/1, ps_s_l/1, Sum/1  "Ts"
  Mux/1 -> wallsurface/1
  Product/1 -> Mux/2, Sum2/3  "qdotr"
  emission_in/1 -> view_factor/1
  Bus Selector/1 -> x2RelHum_UIBK/1, ps_l/1, Mux2/2, Sum/2  "<Tc>"
  AIB/1 -> Bus Selector/1
  Sum2/1 -> qdots/1
  Mux4/1 -> "[S]"/1
  sigma/1 -> emission_in/1
  Mux3/1 -> Fcn1/1
  Fcn1/1 -> Product/2
  x2RelHum_UIBK/1 -> Gain2/1
  Bus Selector/3 -> x2RelHum_UIBK/2  "<p>"
  Bus Selector/4 -> x2RelHum_UIBK/3  "<x_H2O>"
  Gain2/1 -> phi_i_1/100/1, Product2/1
  lewis/1 -> wallsurface1/1
  ps_l/1 -> Product2/2
  ps_s_l/1 -> Product3/2
  Product3/1 -> Add/1
  Product2/1 -> Add/2
  phis/1 -> Switch/2, Product3/1
  view_factor/1 -> Product/1
  wallsurface1/1 -> Switch/1
  Switch/1 -> Mux4/3
  nomassflow/1 -> Switch/3
  Constant5/1 -> Mux4/6
  Constant4/1 -> Mux4/4
  Constant3/1 -> Mux4/2
  Sum of Elements/1 -> Mux4/5
  Product4/1 -> lewis/1
  Add/1 -> Product4/2

== system carnotUIBK/wall_intersection/hygrothermal model/alpha_i1/alpha_i_horizontal ==
  note: dynamic, convective heat transfer coefficients according to: Glück B.: Wärmeübergangskoeffizienten an thermisch aktiven Bauteiloberflächen
      | und der Übergang zu Basiskennlinien für die Wärmestromdichte; gi Gesundheits-Ingenieur; 128. Jahrgang 2007, Heft 1, Seiten 1-10
  note: s: surface
      | c: convective
      | r: radiative
  note: CONVENTION:
      | Qdot > 0 and qdots < 0, if Ts > T (heat flows from wall surface to room node),
      | Qdot < 0 and qdots > 0, if Ts < T (heat flows from room node to wall surface).
  note: Convective and radiative heat transfer at the INDOOR SURFACE of a VERTICAL OUTER WALL
  note: (W/m^2)
  Ts : Inport
  AIB : Inport  Port=2
  Qdot sol : Inport  Port=3
  phis : Inport  Port=4
  1/wallsurface : Gain  Gain=1/wallsurface  SaturateOnIntegerOverflow=on  OutDataTypeStr=Inherit: Same as input  ParamDataTypeStr=Inherit: Same as input
  Add : Sum  Inputs=+-
  Bus Selector : BusSelector  OutputSignals=Tc,Tr,p,x_H2O
  Constant3 : Constant  Value=zeros(1,2)
  Constant4 : Constant  Value=zeros(1,4)
  Constant5 : Constant  Value=zeros(1,9)
  Fcn : Fcn  Expr=1.6*(abs(u(1)-u(2)))^0.3
  Fcn1 : Fcn  Expr=(273.15+u(1))^4-(273.15+u(2))^4
  Gain2 : Gain  Gain=0.01
  Mux : Mux  Inputs=2
  Mux2 : Mux  Inputs=2
  Mux3 : Mux  Inputs=2
  Mux4 : Mux  Inputs=[2 2 1 4 1 9]
  Product : Product  SaturateOnIntegerOverflow=on  RndMeth=Zero  InputSameDT=on  OutDataTypeStr=Inherit: Same as first input
  Product1 : Product  SaturateOnIntegerOverflow=on  RndMeth=Zero  InputSameDT=on  OutDataTypeStr=Inherit: Same as first input
  Product2 : Product  RndMeth=Zero
  Product3 : Product  RndMeth=Zero
  Product4 : Product  SaturateOnIntegerOverflow=on  RndMeth=Zero  InputSameDT=on  OutDataTypeStr=Inherit: Same as first input
  Sum : Sum  Inputs=+-  SaturateOnIntegerOverflow=on  InputSameDT=on  OutDataTypeStr=Inherit: Same as first input
  Sum of Elements : Sum  Inputs=+
  Sum2 : Sum  Inputs=+--  SaturateOnIntegerOverflow=on  InputSameDT=on  OutDataTypeStr=Inherit: Same as first input
  Switch : Switch  Criteria=u2 > Threshold
  emission_in : Gain  Gain=emission_in  SaturateOnIntegerOverflow=on  OutDataTypeStr=Inherit: Same as input  ParamDataTypeStr=Inherit: Same as input
  lewis : Gain  Gain=0.000000007  SaturateOnIntegerOverflow=on  OutDataTypeStr=Inherit: Same as input  ParamDataTypeStr=Inherit: Same as input
  nomassflow : Constant  Value=0
  ps_l : Fcn  Expr=610.0*exp(17.08*(u)/(234.2+(u)))
  ps_s_l : Fcn  Expr=610.0*exp(17.08*(u)/(234.2+(u)))
  sigma : Constant  Value=5.67e-8
  view_factor : Gain  Gain=view_factor  SaturateOnIntegerOverflow=on  OutDataTypeStr=Inherit: Same as input  ParamDataTypeStr=Inherit: Same as input
  wallsurface : Gain  Gain=wallsurface  SaturateOnIntegerOverflow=on  OutDataTypeStr=Inherit: Same as input  ParamDataTypeStr=Inherit: Same as input
  wallsurface1 : Gain  Gain=wallsurface  SaturateOnIntegerOverflow=on  OutDataTypeStr=Inherit: Same as input  ParamDataTypeStr=Inherit: Same as input
  x2RelHum_UIBK : carnot/Basic/Material_Properties/x2RelHum
  qdots : Outport  InitialOutput=0
  "[S]" : Outport  Port=2  InitialOutput=0
  alpha_c : Outport  Port=3  InitialOutput=0
  phi_i_1/100 : Outport  Port=4  InitialOutput=0
  wires:
  1/wallsurface/1 -> Sum2/1
  Qdot sol/1 -> 1/wallsurface/1
  wallsurface/1 -> Sum of Elements/1, Mux4/1  "[Qdotc, Qdotr]"
  Fcn/1 -> Product1/2, Product4/1, alpha_c/1  "hc"
  Product1/1 -> Sum2/2, Mux/1  "qdotc"
  Mux2/1 -> Fcn/1
  Bus Selector/2 -> Mux3/2  "<Tr>"
  Sum/1 -> Product1/1  "dTc"
  Ts/1 -> Mux2/1, Mux3/1, ps_s_l/1, Sum/1  "Ts"
  Mux/1 -> wallsurface/1
  Product/1 -> Mux/2, Sum2/3  "qdotr"
  emission_in/1 -> view_factor/1
  Bus Selector/1 -> x2RelHum_UIBK/1, ps_l/1, Mux2/2, Sum/2  "<Tc>"
  AIB/1 -> Bus Selector/1
  Sum2/1 -> qdots/1
  Mux4/1 -> "[S]"/1
  sigma/1 -> emission_in/1
  Mux3/1 -> Fcn1/1
  Fcn1/1 -> Product/2
  x2RelHum_UIBK/1 -> Gain2/1
  Bus Selector/3 -> x2RelHum_UIBK/2  "<p>"
  Bus Selector/4 -> x2RelHum_UIBK/3  "<x_H2O>"
  Gain2/1 -> phi_i_1/100/1, Product2/1
  lewis/1 -> wallsurface1/1
  ps_l/1 -> Product2/2
  ps_s_l/1 -> Product3/2
  Product3/1 -> Add/1
  Product2/1 -> Add/2
  phis/1 -> Switch/2, Product3/1
  view_factor/1 -> Product/1
  wallsurface1/1 -> Switch/1
  Switch/1 -> Mux4/3
  nomassflow/1 -> Switch/3
  Constant5/1 -> Mux4/6
  Constant4/1 -> Mux4/4
  Constant3/1 -> Mux4/2
  Sum of Elements/1 -> Mux4/5
  Product4/1 -> lewis/1
  Add/1 -> Product4/2

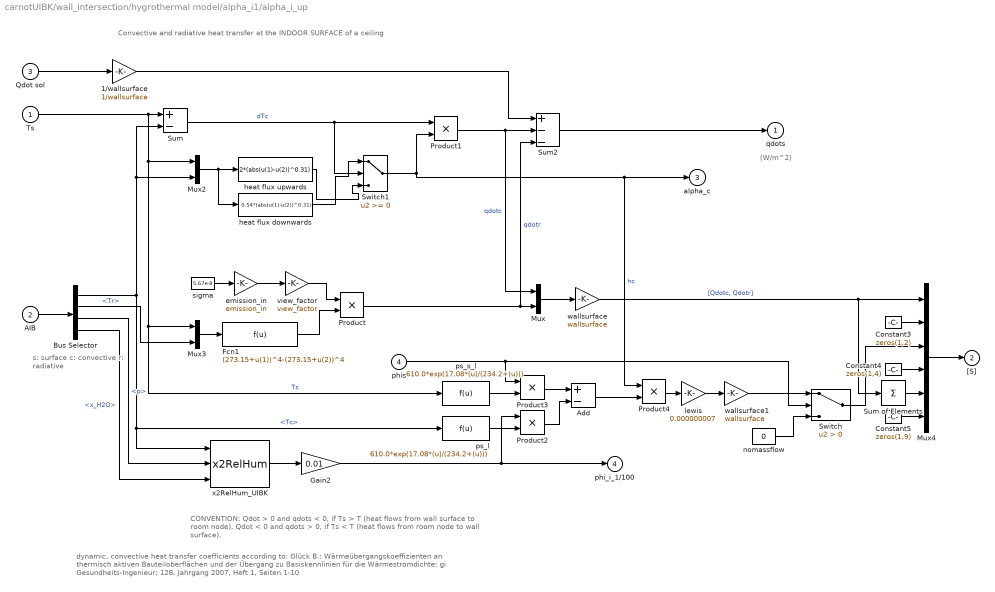
== system carnotUIBK/wall_intersection/hygrothermal model/alpha_i1/alpha_i_up ==
  note: dynamic, convective heat transfer coefficients according to: Glück B.: Wärmeübergangskoeffizienten an thermisch aktiven Bauteiloberflächen
      | und der Übergang zu Basiskennlinien für die Wärmestromdichte; gi Gesundheits-Ingenieur; 128. Jahrgang 2007, Heft 1, Seiten 1-10
  note: s: surface
      | c: convective
      | r: radiative
  note: CONVENTION:
      | Qdot > 0 and qdots < 0, if Ts > T (heat flows from wall surface to room node),
      | Qdot < 0 and qdots > 0, if Ts < T (heat flows from room node to wall surface).
  note: Convective and radiative heat transfer at the INDOOR SURFACE of a ceiling
  note: (W/m^2)
  Ts : Inport
  AIB : Inport  Port=2
  Qdot sol : Inport  Port=3
  phis : Inport  Port=4
  1/wallsurface : Gain  Gain=1/wallsurface  SaturateOnIntegerOverflow=on  OutDataTypeStr=Inherit: Same as input  ParamDataTypeStr=Inherit: Same as input
  Add : Sum  Inputs=+-
  Bus Selector : BusSelector  OutputSignals=Tc,Tr,p,x_H2O
  Constant3 : Constant  Value=zeros(1,2)
  Constant4 : Constant  Value=zeros(1,4)
  Constant5 : Constant  Value=zeros(1,9)
  Fcn1 : Fcn  Expr=(273.15+u(1))^4-(273.15+u(2))^4
  Gain2 : Gain  Gain=0.01
  Mux : Mux  Inputs=2
  Mux2 : Mux  Inputs=2
  Mux3 : Mux  Inputs=2
  Mux4 : Mux  Inputs=[2 2 1 4 1 9]
  Product : Product  SaturateOnIntegerOverflow=on  RndMeth=Zero  InputSameDT=on  OutDataTypeStr=Inherit: Same as first input
  Product1 : Product  SaturateOnIntegerOverflow=on  RndMeth=Zero  InputSameDT=on  OutDataTypeStr=Inherit: Same as first input
  Product2 : Product  RndMeth=Zero
  Product3 : Product  RndMeth=Zero
  Product4 : Product  SaturateOnIntegerOverflow=on  RndMeth=Zero  InputSameDT=on  OutDataTypeStr=Inherit: Same as first input
  Sum : Sum  Inputs=+-  SaturateOnIntegerOverflow=on  InputSameDT=on  OutDataTypeStr=Inherit: Same as first input
  Sum of Elements : Sum  Inputs=+
  Sum2 : Sum  Inputs=+--  SaturateOnIntegerOverflow=on  InputSameDT=on  OutDataTypeStr=Inherit: Same as first input
  Switch : Switch  Criteria=u2 > Threshold
  Switch1 : Switch
  emission_in : Gain  Gain=emission_in  SaturateOnIntegerOverflow=on  OutDataTypeStr=Inherit: Same as input  ParamDataTypeStr=Inherit: Same as input
  heat flux downwards : Fcn  Expr=0.54*(abs(u(1)-u(2))^0.31)
  heat flux upwards : Fcn  Expr=2*(abs(u(1)-u(2))^0.31)
  lewis : Gain  Gain=0.000000007  SaturateOnIntegerOverflow=on  OutDataTypeStr=Inherit: Same as input  ParamDataTypeStr=Inherit: Same as input
  nomassflow : Constant  Value=0
  ps_l : Fcn  Expr=610.0*exp(17.08*(u)/(234.2+(u)))
  ps_s_l : Fcn  Expr=610.0*exp(17.08*(u)/(234.2+(u)))
  sigma : Constant  Value=5.67e-8
  view_factor : Gain  Gain=view_factor  SaturateOnIntegerOverflow=on  OutDataTypeStr=Inherit: Same as input  ParamDataTypeStr=Inherit: Same as input
  wallsurface : Gain  Gain=wallsurface  SaturateOnIntegerOverflow=on  OutDataTypeStr=Inherit: Same as input  ParamDataTypeStr=Inherit: Same as input
  wallsurface1 : Gain  Gain=wallsurface  SaturateOnIntegerOverflow=on  OutDataTypeStr=Inherit: Same as input  ParamDataTypeStr=Inherit: Same as input
  x2RelHum_UIBK : carnot/Basic/Material_Properties/x2RelHum
  qdots : Outport  InitialOutput=0
  "[S]" : Outport  Port=2  InitialOutput=0
  alpha_c : Outport  Port=3  InitialOutput=0
  phi_i_1/100 : Outport  Port=4  InitialOutput=0
  wires:
  heat flux downwards/1 -> Switch1/1
  heat flux upwards/1 -> Switch1/3
  Sum/1 -> Product1/1, Switch1/2  "dTc"
  1/wallsurface/1 -> Sum2/1
  Qdot sol/1 -> 1/wallsurface/1
  wallsurface/1 -> Sum of Elements/1, Mux4/1  "[Qdotc, Qdotr]"
  Switch1/1 -> Product4/1, alpha_c/1, Product1/2  "hc"
  Product1/1 -> Sum2/2, Mux/1  "qdotc"
  Mux2/1 -> heat flux upwards/1, heat flux downwards/1
  Bus Selector/2 -> Mux3/2  "<Tr>"
  Ts/1 -> Mux2/1, Mux3/1, ps_s_l/1, Sum/1  "Ts"
  Mux/1 -> wallsurface/1
  Product/1 -> Mux/2, Sum2/3  "qdotr"
  emission_in/1 -> view_factor/1
  Bus Selector/1 -> x2RelHum_UIBK/1, ps_l/1, Mux2/2, Sum/2  "<Tc>"
  AIB/1 -> Bus Selector/1
  Sum2/1 -> qdots/1
  Switch/1 -> Mux4/3
  sigma/1 -> emission_in/1
  Mux3/1 -> Fcn1/1
  Fcn1/1 -> Product/2
  x2RelHum_UIBK/1 -> Gain2/1
  Bus Selector/3 -> x2RelHum_UIBK/2  "<p>"
  Bus Selector/4 -> x2RelHum_UIBK/3  "<x_H2O>"
  Gain2/1 -> phi_i_1/100/1, Product2/1
  lewis/1 -> wallsurface1/1
  ps_l/1 -> Product2/2
  ps_s_l/1 -> Product3/2
  Product3/1 -> Add/1
  Product2/1 -> Add/2
  phis/1 -> Switch/2, Product3/1
  view_factor/1 -> Product/1
  wallsurface1/1 -> Switch/1
  nomassflow/1 -> Switch/3
  Constant5/1 -> Mux4/6
  Constant4/1 -> Mux4/4
  Constant3/1 -> Mux4/2
  Sum of Elements/1 -> Mux4/5
  Mux4/1 -> "[S]"/1
  Product4/1 -> lewis/1
  Add/1 -> Product4/2

== system carnotUIBK/wall_intersection/hygrothermal model/alpha_i2/alpha_i_down ==
  note: (W/m^2)
  note: Convective and radiative heat transfer at the INDOOR SURFACE of a floor
  note: CONVENTION:
      | Qdot > 0 and qdots < 0, if Ts > T (heat flows from wall surface to room node),
      | Qdot < 0 and qdots > 0, if Ts < T (heat flows from room node to wall surface).
  note: s: surface
      | c: convective
      | r: radiative
  note: dynamic, convective heat transfer coefficients according to: Glück B.: Wärmeübergangskoeffizienten an thermisch aktiven Bauteiloberflächen
      | und der Übergang zu Basiskennlinien für die Wärmestromdichte; gi Gesundheits-Ingenieur; 128. Jahrgang 2007, Heft 1, Seiten 1-10
  Ts : Inport
  AIB : Inport  Port=2
  Qdot sol : Inport  Port=3
  phis : Inport  Port=4
  1/wallsurface : Gain  Gain=1/wallsurface  SaturateOnIntegerOverflow=on  OutDataTypeStr=Inherit: Same as input  ParamDataTypeStr=Inherit: Same as input
  Add : Sum  Inputs=+-
  Bus Selector : BusSelector  OutputSignals=Tc,Tr,p,x_H2O
  Constant3 : Constant  Value=zeros(1,2)
  Constant4 : Constant  Value=zeros(1,4)
  Constant5 : Constant  Value=zeros(1,9)
  Fcn1 : Fcn  Expr=(273.15+u(1))^4-(273.15+u(2))^4
  Gain2 : Gain  Gain=0.01
  Mux : Mux  Inputs=2
  Mux2 : Mux  Inputs=2
  Mux3 : Mux  Inputs=2
  Mux4 : Mux  Inputs=[2 2 1 4 1 9]
  Product : Product  SaturateOnIntegerOverflow=on  RndMeth=Zero  InputSameDT=on  OutDataTypeStr=Inherit: Same as first input
  Product1 : Product  SaturateOnIntegerOverflow=on  RndMeth=Zero  InputSameDT=on  OutDataTypeStr=Inherit: Same as first input
  Product2 : Product  RndMeth=Zero
  Product3 : Product  RndMeth=Zero
  Product4 : Product  SaturateOnIntegerOverflow=on  RndMeth=Zero  InputSameDT=on  OutDataTypeStr=Inherit: Same as first input
  Sum : Sum  Inputs=+-  SaturateOnIntegerOverflow=on  InputSameDT=on  OutDataTypeStr=Inherit: Same as first input
  Sum of Elements : Sum  Inputs=+
  Sum2 : Sum  Inputs=+--  SaturateOnIntegerOverflow=on  InputSameDT=on  OutDataTypeStr=Inherit: Same as first input
  Switch : Switch  Criteria=u2 > Threshold
  Switch1 : Switch
  emission_in : Gain  Gain=emission_in  SaturateOnIntegerOverflow=on  OutDataTypeStr=Inherit: Same as input  ParamDataTypeStr=Inherit: Same as input
  heat flux downwards : Fcn  Expr=0.54*(abs(u(1)-u(2))^0.31)
  heat flux upwards : Fcn  Expr=2*(abs(u(1)-u(2))^0.31)
  lewis : Gain  Gain=0.000000007  SaturateOnIntegerOverflow=on  OutDataTypeStr=Inherit: Same as input  ParamDataTypeStr=Inherit: Same as input
  nomassflow : Constant  Value=0
  ps_l : Fcn  Expr=610.0*exp(17.08*(u)/(234.2+(u)))
  ps_s_l : Fcn  Expr=610.0*exp(17.08*(u)/(234.2+(u)))
  sigma : Constant  Value=5.67e-8
  view_factor : Gain  Gain=view_factor  SaturateOnIntegerOverflow=on  OutDataTypeStr=Inherit: Same as input  ParamDataTypeStr=Inherit: Same as input
  wallsurface : Gain  Gain=wallsurface  SaturateOnIntegerOverflow=on  OutDataTypeStr=Inherit: Same as input  ParamDataTypeStr=Inherit: Same as input
  wallsurface1 : Gain  Gain=wallsurface  SaturateOnIntegerOverflow=on  OutDataTypeStr=Inherit: Same as input  ParamDataTypeStr=Inherit: Same as input
  x2RelHum_UIBK : carnot/Basic/Material_Properties/x2RelHum
  qdots : Outport  InitialOutput=0
  "[S]" : Outport  Port=2  InitialOutput=0
  alpha_c : Outport  Port=3  InitialOutput=0
  phi_i_1/100 : Outport  Port=4  InitialOutput=0
  wires:
  nomassflow/1 -> Switch/3
  Switch/1 -> Mux4/3
  wallsurface1/1 -> Switch/1
  view_factor/1 -> Product/1
  phis/1 -> Product3/1, Switch/2
  Product2/1 -> Add/2
  Product3/1 -> Add/1
  ps_s_l/1 -> Product3/2
  ps_l/1 -> Product2/2
  lewis/1 -> wallsurface1/1
  Gain2/1 -> Product2/1, phi_i_1/100/1
  Bus Selector/4 -> x2RelHum_UIBK/3  "<x_H2O>"
  Bus Selector/3 -> x2RelHum_UIBK/2  "<p>"
  x2RelHum_UIBK/1 -> Gain2/1
  Fcn1/1 -> Product/2
  Mux3/1 -> Fcn1/1
  sigma/1 -> emission_in/1
  Mux4/1 -> "[S]"/1
  Sum2/1 -> qdots/1
  AIB/1 -> Bus Selector/1
  Bus Selector/1 -> Sum/2, Mux2/2, x2RelHum_UIBK/1, ps_l/1  "<Tc>"
  emission_in/1 -> view_factor/1
  Product/1 -> Sum2/3, Mux/2  "qdotr"
  Mux/1 -> wallsurface/1
  Ts/1 -> Sum/1, ps_s_l/1, Mux3/1, Mux2/1  "Ts"
  Bus Selector/2 -> Mux3/2  "<Tr>"
  Mux2/1 -> heat flux downwards/1, heat flux upwards/1
  Product1/1 -> Mux/1, Sum2/2  "qdotc"
  Switch1/1 -> Product1/2, Product4/1, alpha_c/1  "hc"
  wallsurface/1 -> Sum of Elements/1, Mux4/1  "[Qdotc, Qdotr]"
  Qdot sol/1 -> 1/wallsurface/1
  1/wallsurface/1 -> Sum2/1
  Sum/1 -> Switch1/2, Product1/1  "dTc"
  heat flux upwards/1 -> Switch1/1
  heat flux downwards/1 -> Switch1/3
  Constant5/1 -> Mux4/6
  Constant4/1 -> Mux4/4
  Constant3/1 -> Mux4/2
  Sum of Elements/1 -> Mux4/5
  Product4/1 -> lewis/1
  Add/1 -> Product4/2
